simulink model "LQG_24aprile"  (R2025b)
settings: Solver=VariableStepAuto  StartTime=0.0  StopTime=30.0  RelTol=1e-3
undefined symbols (not defined in the file): A, B, C, G, K_LQR_i, K_LQR_x, Qv, Rv, Ts_lqr, x0_lmi, xref_lqg
libraries: cstblocks x1
settings Model: Creator=salvo  LastModifiedBy=salvo

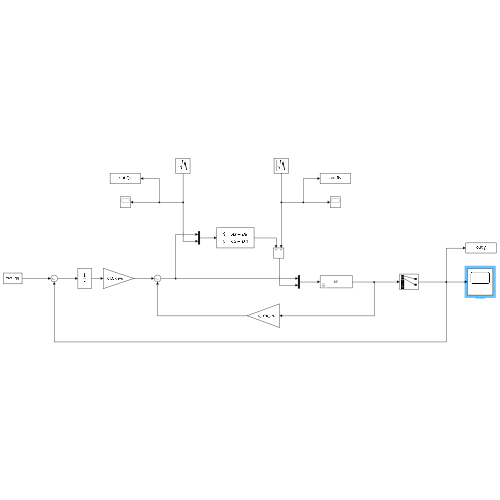
[thumbnail: Simulink's stored preview of the top-level diagram]
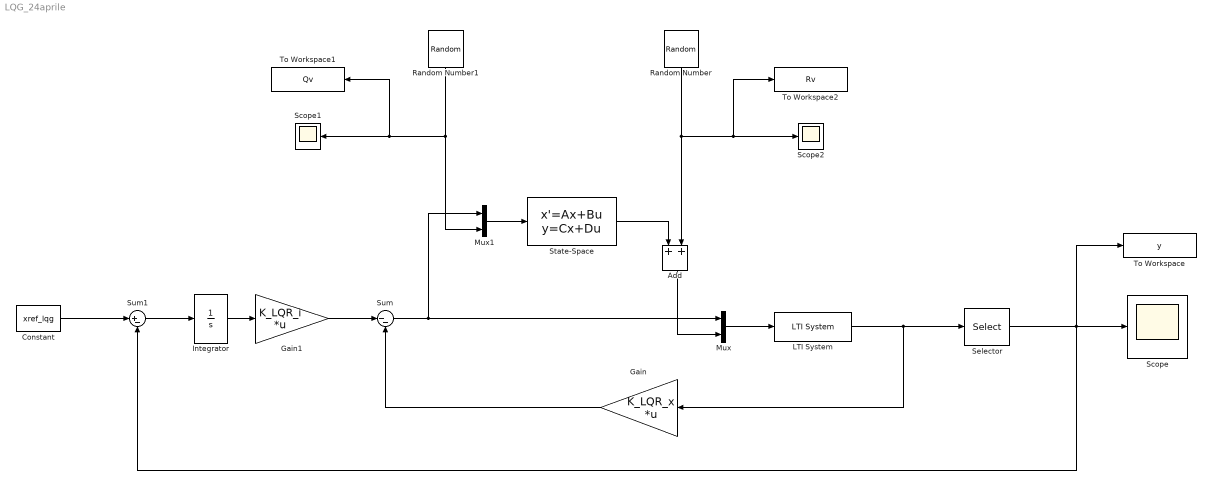
== system LQG_24aprile ==
  Add : Sum
  Constant : Constant  Value=xref_lqg
  Gain : Gain  Gain=K_LQR_x  Multiplication=Matrix(K*u)
  Gain1 : Gain  Gain=K_LQR_i  Multiplication=Matrix(K*u)
  Integrator : Integrator
  LTI System : cstblocks/LTI System  sys=KF  IC=[]  PadeOrder=0
  Mux : Mux  Inputs=2
  Mux1 : Mux  Inputs=2
  Random Number : RandomNumber  Variance=diag(Rv)  SampleTime=Ts_lqr
  Random Number1 : RandomNumber  Variance=diag(Qv)  SampleTime=Ts_lqr
  Scope : Scope
      settings: ActiveDisplayYMinimum=-42.282610978506625  ActiveDisplayYMaximum=35.606253050639147
  Scope1 : Scope
      settings: ActiveDisplayYMinimum=-1  ActiveDisplayYMaximum=1
  Scope2 : Scope
      settings: ActiveDisplayYMinimum=-1  ActiveDisplayYMaximum=1  DataLoggingVariableName=ScopeData2
  Selector : Selector  InputPortWidth=6  IndexOptions=Index vector (dialog)  Indices=[1 2]  OutputSizes=1
  State-Space : StateSpace  A=A  B=[B G]  C=C(1:2,:)  D=zeros(2,8)  InitialCondition=x0_lmi
  Sum : Sum  Inputs=|--
  Sum1 : Sum  Inputs=|+-
  To Workspace : ToWorkspace  VariableName=y  SaveFormat=Timeseries  SampleTime=-1
  To Workspace1 : ToWorkspace  VariableName=Qv  SaveFormat=Timeseries  SampleTime=-1
  To Workspace2 : ToWorkspace  VariableName=Rv  SaveFormat=Timeseries  SampleTime=-1
  wires:
  Integrator/1 -> Gain1/1
  Gain1/1 -> Sum/1
  Gain/1 -> Sum/2
  Selector/1 -> To Workspace/1, Scope/1, Sum1/2
  Sum1/1 -> Integrator/1
  Constant/1 -> Sum1/1
  Sum/1 -> Mux1/1, Mux/1
  Mux/1 -> LTI System/1
  LTI System/1 -> Selector/1, Gain/1
  Random Number/1 -> To Workspace2/1, Scope2/1, Add/2
  State-Space/1 -> Add/1
  Mux1/1 -> State-Space/1
  Random Number1/1 -> Mux1/2, To Workspace1/1, Scope1/1
  Add/1 -> Mux/2
